simulink model "CAProcessorInTheLoop"  (R2022b)
settings: Solver=FixedStepAuto  StartTime=0.0  StopTime=100.0  RelTol=1e-3  EnableMultiTasking=on
InitFcn:
  | init_fn()
values from neighbouring files (symbols this model uses):
  X_air = evalin('base', 'X_air')    [init_fn.m]
undefined symbols (not defined in the file or in its folder): m, MAX_SPEED_BACKWARD, MAX_SPEED_FORWARD, MAX_TORQUE, MAX_TORQUE_REVERSE, r, TRANSMISSION_RATIO, X_tyres
libraries: arduinolib x25, slpidlib x1
settings Model: ExtModeTrigDuration=2  Creator=David  LastModifiedBy=David
settings OptimizationCC: EnhancedBackFolding=on  PassReuseOutputArgsAs=Individual arguments  ZeroExternalMemoryAtStartup=off  ZeroInternalMemoryAtStartup=off  MaxStackSize=64  OptimizeBlockOrder=speed  DifferentSizesBufferReuse=on  OptimizationCustomize=off  EfficientTunableParamExpr=on
settings DebuggingCC: ParameterOverflowMsg=none  ParameterUnderflowMsg=error  ParameterPrecisionLossMsg=none  ParameterTunabilityLossMsg=error
settings HardwareCC: ProdBitPerInt=16  ProdBitPerPointer=16  ProdBitPerSizeT=16  ProdBitPerPtrDiffT=16  ProdLargestAtomicFloat=None  ProdWordSize=8  ProdHWDeviceType=Atmel->AVR
settings SFSimCC: MATLABDynamicMemAlloc=off
settings RTWCC: Description=Embedded Coder  SystemTargetFile=ert.tlc  HardwareBoard=Arduino Mega 2560  TLCOptions=-aInlineSetEventsForThisBaseRateFcn=TLC_FALSE -aSuppressMultiTaskScheduler=TLC_FALSE -aRateBasedStepFcn=1  TemplateMakefile=ert_default_tmf  Toolchain=Arduino AVR
settings CodeAppCC: ForceParamTrailComments=on  IgnoreCustomStorageClasses=off  OperatorAnnotations=on  SimulinkDataObjDesc=on  SFDataObjDesc=on  InsertBlockDesc=on
settings ERTTargetCC: SupportContinuousTime=on  SupportVariableSizeSignals=on  ExtModeTransport=3  ExtModeStaticAlloc=on  ExtModeAutomaticAllocSize=off  ExtModeStaticAllocSize=2048  ExtModeMexFile=ext_xcp  ExtModeIntrfLevel=Level2 - Open

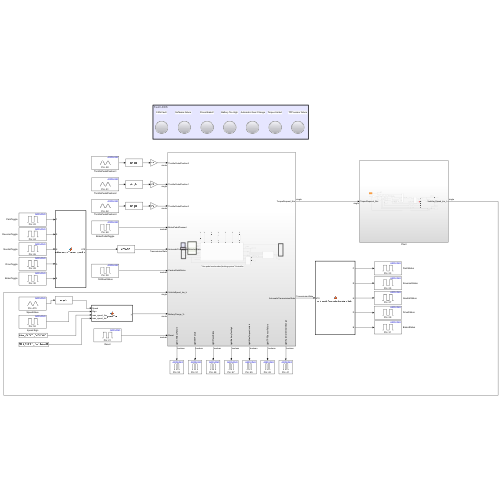
[thumbnail: Simulink's stored preview of the top-level diagram]
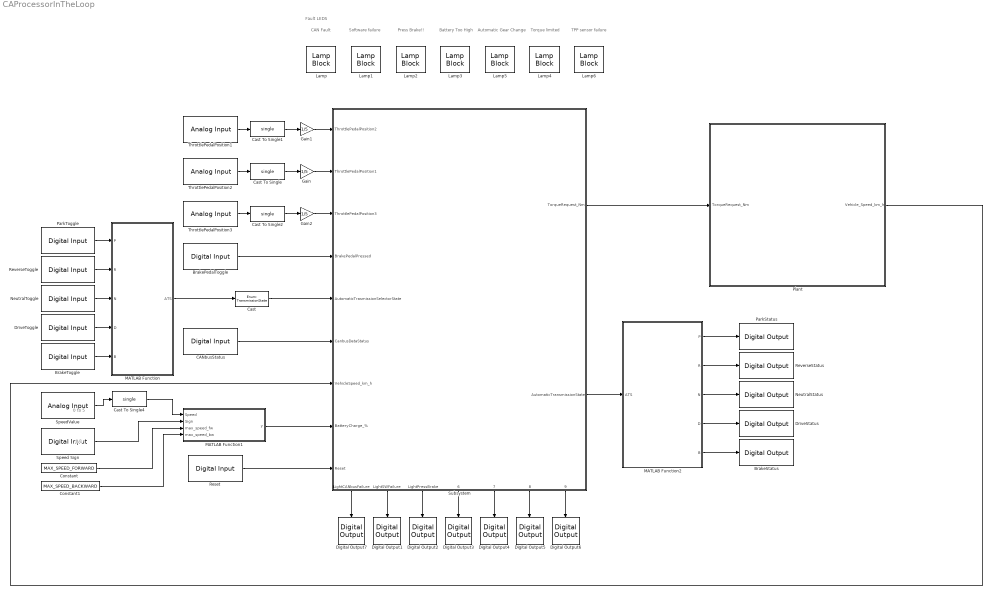
== system CAProcessorInTheLoop ==
  note: Fault LEDS
  note: 0 to 5
  note: CAN Fault
  note: Automatic Gear Change
  note: Press Brake!!
  note: Battery Too High
  note: Software failure
  note: TPP sensor failure
  note: Torque limited
  note: 0/1
  BrakePedalToggle : arduinolib/Digital Input  pinNumber=48  mode=Default  Direction=input  SampleTime=0.01  blockPlatform=arduino
  BrakeStatus : arduinolib/Digital Output  pinNumber=31  Direction=output  blockPlatform=arduino
  BrakeToggle : arduinolib/Digital Input  pinNumber=30  mode=Default  Direction=input  SampleTime=0.01  blockPlatform=arduino
  CANbusStatus : arduinolib/Digital Input  pinNumber=50  mode=Default  Direction=input  SampleTime=0.01  blockPlatform=arduino
  Cast : DataTypeConversion  OutDataTypeStr=Enum: TransmissionState  SaturateOnIntegerOverflow=off  RndMeth=Floor
  Cast To Single{,1..2,4} (4 alike) : DataTypeConversion  OutDataTypeStr=single  SaturateOnIntegerOverflow=off  RndMeth=Floor
  Constant : Constant  Value=MAX_SPEED_FORWARD  OutDataTypeStr=single
  Constant1 : Constant  Value=MAX_SPEED_BACKWARD  OutDataTypeStr=single
  Digital Output1 : arduinolib/Digital Output  pinNumber=51  Direction=output  blockPlatform=arduino
  Digital Output2 : arduinolib/Digital Output  pinNumber=49  Direction=output  blockPlatform=arduino
  Digital Output3 : arduinolib/Digital Output  pinNumber=47  Direction=output  blockPlatform=arduino
  Digital Output4 : arduinolib/Digital Output  pinNumber=45  Direction=output  blockPlatform=arduino
  Digital Output5 : arduinolib/Digital Output  pinNumber=43  Direction=output  blockPlatform=arduino
  Digital Output6 : arduinolib/Digital Output  pinNumber=41  Direction=output  blockPlatform=arduino
  Digital Output7 : arduinolib/Digital Output  pinNumber=53  Direction=output  blockPlatform=arduino
  DriveStatus : arduinolib/Digital Output  pinNumber=29  Direction=output  blockPlatform=arduino
  DriveToggle : arduinolib/Digital Input  pinNumber=28  mode=Default  Direction=input  SampleTime=0.01  blockPlatform=arduino
  Gain : Gain  Gain=1/5
  Gain1 : Gain  Gain=1/5
  Gain2 : Gain  Gain=1/5
  Lamp{,1..6} (7 alike) : LampBlock  LabelPosition=Hide
  MATLAB Function : MATLAB Function  TreatAsAtomicUnit=on
  MATLAB Function1 : MATLAB Function  TreatAsAtomicUnit=on
  MATLAB Function2 : MATLAB Function  TreatAsAtomicUnit=on
  NeutralStatus : arduinolib/Digital Output  pinNumber=27  Direction=output  blockPlatform=arduino
  NeutralToggle : arduinolib/Digital Input  pinNumber=26  mode=Default  Direction=input  SampleTime=0.01  blockPlatform=arduino
  ParkStatus : arduinolib/Digital Output  pinNumber=23  Direction=output  blockPlatform=arduino
  ParkToggle : arduinolib/Digital Input  pinNumber=22  mode=Default  Direction=input  SampleTime=0.01  blockPlatform=arduino
  Plant : Subsystem
  Reset : arduinolib/Digital Input  pinNumber=21  mode=Default  Direction=input  SampleTime=0.01  blockPlatform=arduino
  ReverseStatus : arduinolib/Digital Output  pinNumber=25  Direction=output  blockPlatform=arduino
  ReverseToggle : arduinolib/Digital Input  pinNumber=24  mode=Default  Direction=input  SampleTime=0.01  blockPlatform=arduino
  Speed Sign : arduinolib/Digital Input  pinNumber=52  mode=Default  Direction=input  SampleTime=0.01  blockPlatform=arduino
  SpeedValue : arduinolib/Analog Input  pinNumber=15  ReadResultsOnly=off  ConversionTriggerSource=Software  ExternalTriggerType=uint32( 0 )  OutputDataType=uint16  EnableConversionCompleteNotify=off  EnableOuputStatus=off  SampleTime=-1  blockPlatform=arduino
  Subsystem : Subsystem
      settings: PortSchema="{\"entries\":[{\"content\":{\"sides\":[{\"content\":{\"connectorIds\":[\"In1\",\"In2\",\"In3\",\"In4\",\"In5\",\"In6\",\"In7\",\"In8\",\"In9\"]},\"type\":\"ConnectorPlacement.EquallySpacedRectSide\",\"uuid\":\"240cc9ec-2ba8-4d42-9768-bf8b5b2cd18c\"},{\"content\":{\"connectorIds\":[\"Out1\",\"Out2\"],\"side\":\"RIGHT\"},\"type\":\"ConnectorPlacement.EquallySpacedRectSide\",\"uuid\":\"79e5a8d1-1f90-4926-ab4a-0fddf072b8d0\"},{\"content\":{\"connectorIds\":[],\"side\":\"TOP\"},\"type\":\"ConnectorPlacement.EquallySpacedRectSide\",\"uuid\":\"0e8827e4-c087-4ef4-9de2-35b882084602\"},{\"content\":{\"connectorIds\":[\"Out3\",\"Out4\",\"Out5\",\"Out6\",\"Out7\",\"Out8\",\"Out9\"],\"side\":\"BOTTOM\"},\"type\":\"ConnectorPlacement.EquallySpacedRectSide\",\"uuid\":\"1cd7cba7-84b1-4c6c-afc4-562411f8f962\"}]},\"type\":\"ConnectorPlacement.EquallySpacedConnector\",\"uuid\":\"eda7bf13-88b7-423b-9505-3784a3aa3e13\"}],\"packageUris\":[\"http://schema.mathworks.com/mf0/Connector/R2020b\"],\"version\":\"1.0\"}"
  ThrottlePedalPosition1 : arduinolib/Analog Input  pinNumber=0  ReadResultsOnly=off  ConversionTriggerSource=Software  ExternalTriggerType=uint32( 0 )  OutputDataType=uint16  EnableConversionCompleteNotify=off  EnableOuputStatus=off  SampleTime=-1  blockPlatform=arduino
  ThrottlePedalPosition2 : arduinolib/Analog Input  pinNumber=1  ReadResultsOnly=off  ConversionTriggerSource=Software  ExternalTriggerType=uint32( 0 )  OutputDataType=uint16  EnableConversionCompleteNotify=off  EnableOuputStatus=off  SampleTime=-1  blockPlatform=arduino
  ThrottlePedalPosition3 : arduinolib/Analog Input  pinNumber=2  ReadResultsOnly=off  ConversionTriggerSource=Software  ExternalTriggerType=uint32( 0 )  OutputDataType=uint16  EnableConversionCompleteNotify=off  EnableOuputStatus=off  SampleTime=-1  blockPlatform=arduino
  wires:
  ThrottlePedalPosition2/1 -> Cast To Single/1
  Gain/1 -> Subsystem/2(ThrottlePedalPosition1)
  Gain1/1 -> Subsystem/1(ThrottlePedalPosition2)
  ThrottlePedalPosition1/1 -> Cast To Single1/1
  Gain2/1 -> Subsystem/3(ThrottlePedalPosition3)
  ThrottlePedalPosition3/1 -> Cast To Single2/1
  ParkToggle/1 -> MATLAB Function/1(P)
  ReverseToggle/1 -> MATLAB Function/2(R)
  NeutralToggle/1 -> MATLAB Function/3(N)
  DriveToggle/1 -> MATLAB Function/4(D)
  CANbusStatus/1 -> Subsystem/6(CanbusDataStatus)
  SpeedValue/1 -> Cast To Single4/1
  MATLAB Function1/1(y) -> Subsystem/8(BatteryCharge_%)
  Speed Sign/1 -> MATLAB Function1/2(Sign)
  Subsystem/2(AutomaticTransmissionState) -> MATLAB Function2/1(ATS)
  MATLAB Function2/1(P) -> ParkStatus/1
  MATLAB Function2/2(R) -> ReverseStatus/1
  MATLAB Function2/3(N) -> NeutralStatus/1
  MATLAB Function2/4(D) -> DriveStatus/1
  MATLAB Function2/5(B) -> BrakeStatus/1
  Subsystem/1(TorqueRequest_Nm) -> Plant/1(TorqueRequest_Nm)
  Cast To Single/1 -> Gain/1
  Cast To Single1/1 -> Gain1/1
  Cast To Single2/1 -> Gain2/1
  Cast To Single4/1 -> MATLAB Function1/1(Speed)
  Constant/1 -> MATLAB Function1/3(max_speed_fw)
  Constant1/1 -> MATLAB Function1/4(max_speed_bw)
  Cast/1 -> Subsystem/5(AutomaticTrasmissionSelectorState)
  MATLAB Function/1(ATS) -> Cast/1
  BrakePedalToggle/1 -> Subsystem/4(BrakePedalPressed)
  BrakeToggle/1 -> MATLAB Function/5(B)
  Subsystem/3(LightCANbusFailure) -> Digital Output7/1
  Subsystem/4(LightSWFailure) -> Digital Output1/1
  Subsystem/5(LightPressBrake) -> Digital Output2/1
  Subsystem/6(LightBatteryTooHigh) -> Digital Output3/1
  Subsystem/7(LightMaxTorqueLimited) -> Digital Output4/1
  Subsystem/8(LightTPPSensorFailure) -> Digital Output5/1
  Subsystem/9(LightAutomaticGearChange) -> Digital Output6/1
  Reset/1 -> Subsystem/9(Reset)
  Plant/1(Vehicle_Speed_km_h) -> Subsystem/7(VehicleSpeed_km_h)

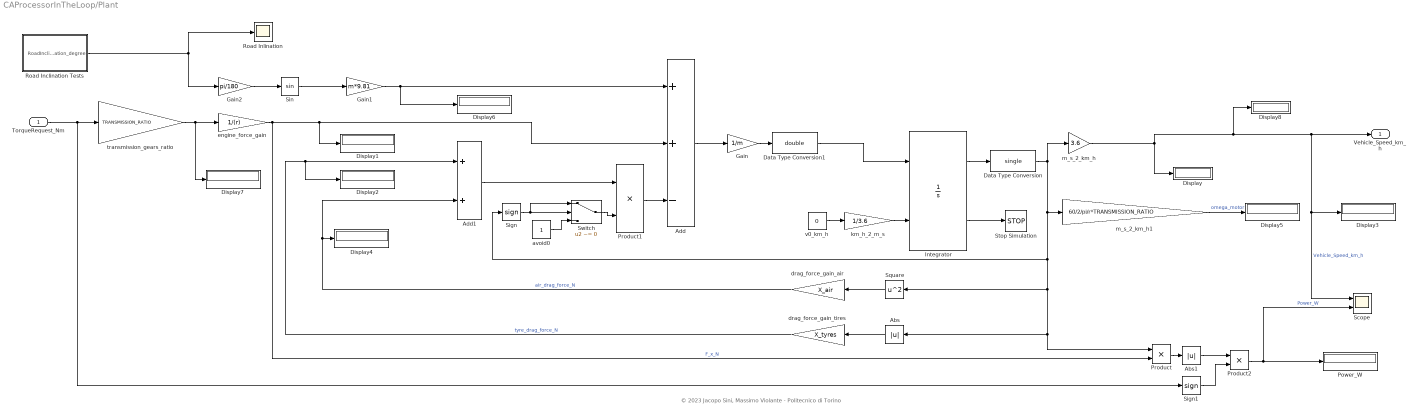
== system CAProcessorInTheLoop/Plant ==
  note: © 2023 Jacopo Sini, Massimo Violante - Politecnico di Torino
  TorqueRequest_Nm : Inport  OutDataTypeStr=single
  Abs : Abs  SaturateOnIntegerOverflow=off
  Abs1 : Abs  SaturateOnIntegerOverflow=off
  Add : Sum  Inputs=++-
  Add1 : Sum
  Data Type Conversion : DataTypeConversion  OutDataTypeStr=single  SaturateOnIntegerOverflow=off  RndMeth=Floor  LockScale=on
  Data Type Conversion1 : DataTypeConversion  OutDataTypeStr=double  SaturateOnIntegerOverflow=off  RndMeth=Floor  LockScale=on
  Display{,1..8} (9 alike) : Display
      Display1 settings: Format=bank
      Display2 settings: Format=bank
      Display3 settings: Format=bank
      Display4 settings: Format=bank
      Display5 settings: Format=bank
      Display6 settings: Format=bank
      Display7 settings: Format=bank
  Gain : Gain  Gain=1/m
  Gain1 : Gain  Gain=m*9.81
  Gain2 : Gain  Gain=pi/180
  Integrator : Integrator  InitialConditionSource=external  LimitOutput=on  UpperSaturationLimit=MAX_SPEED_FORWARD/3.6  LowerSaturationLimit=-MAX_SPEED_BACKWARD/3.6  ShowSaturationPort=on  ContinuousStateAttributes='vehicle_speed'
  Power_W : Display
      settings: Format=bank
  Product : Product
  Product1 : Product
  Product2 : Product
  Road Inclination Tests : Subsystem
  Road Inlination : Scope
  Scope : Scope  NumInputPorts=2
  Sign : Signum  ZeroCross=off
  Sign1 : Signum  ZeroCross=off
  Sin : Trigonometry  OutputSignalType=real
  Square : Math  Operator=square
  Stop Simulation : Stop
  Switch : Switch  Criteria=u2 ~= 0  SaturateOnIntegerOverflow=off  InputSameDT=off
  avoid0 : Constant  OutDataTypeStr=double
  drag_force_gain_air : Gain  Gain=X_air
  drag_force_gain_tires : Gain  Gain=X_tyres
  engine_force_gain : Gain  Gain=1/(r)
  km_h_2_m_s : Gain  Gain=1/3.6
  m_s_2_km_h : Gain  Gain=3.6
  m_s_2_km_h1 : Gain  Gain=60/2/pi/r*TRANSMISSION_RATIO
  transmission_gears_ratio : Gain  Gain=TRANSMISSION_RATIO
  v0_km_h : Constant  Value=0  OutDataTypeStr=double
  Vehicle_Speed_km_h : Outport  OutDataTypeStr=single  Unit=km/h
  wires:
  TorqueRequest_Nm/1 -> Sign1/1, transmission_gears_ratio/1
  Add1/1 -> Product1/1
  Square/1 -> drag_force_gain_air/1
  Data Type Conversion1/1 -> Integrator/1
  v0_km_h/1 -> km_h_2_m_s/1
  Product1/1 -> Add/3
  engine_force_gain/1 -> Product/2, Display1/1, Add/2  "F_x_N"
  Sign/1 -> Switch/1, Switch/2
  Abs/1 -> drag_force_gain_tires/1
  Sign1/1 -> Product2/2
  Abs1/1 -> Product2/1
  km_h_2_m_s/1 -> Integrator/2
  Gain1/1 -> Display6/1, Add/1
  Product2/1 -> Scope/2, Power_W/1  "Power_W"
  Integrator/1 -> Data Type Conversion/1
  drag_force_gain_tires/1 -> Display2/1, Add1/1  "tyre_drag_force_N"
  Sin/1 -> Gain1/1
  Product/1 -> Abs1/1
  Data Type Conversion/1 -> Sign/1, Product/1, Abs/1, Square/1, m_s_2_km_h1/1, m_s_2_km_h/1
  transmission_gears_ratio/1 -> engine_force_gain/1, Display7/1
  avoid0/1 -> Switch/3
  Switch/1 -> Product1/2
  Road Inclination Tests/1(RoadInclination_degree) -> Road Inlination/1, Gain2/1
  Gain2/1 -> Sin/1
  drag_force_gain_air/1 -> Add1/2, Display4/1  "air_drag_force_N"
  Gain/1 -> Data Type Conversion1/1
  Add/1 -> Gain/1
  m_s_2_km_h/1 -> Display8/1, Scope/1, Display3/1, Vehicle_Speed_km_h/1, Display/1  "Vehicle_Speed_km_h"
  Integrator/2 -> Stop Simulation/1
  m_s_2_km_h1/1 -> Display5/1  "omega_motor"

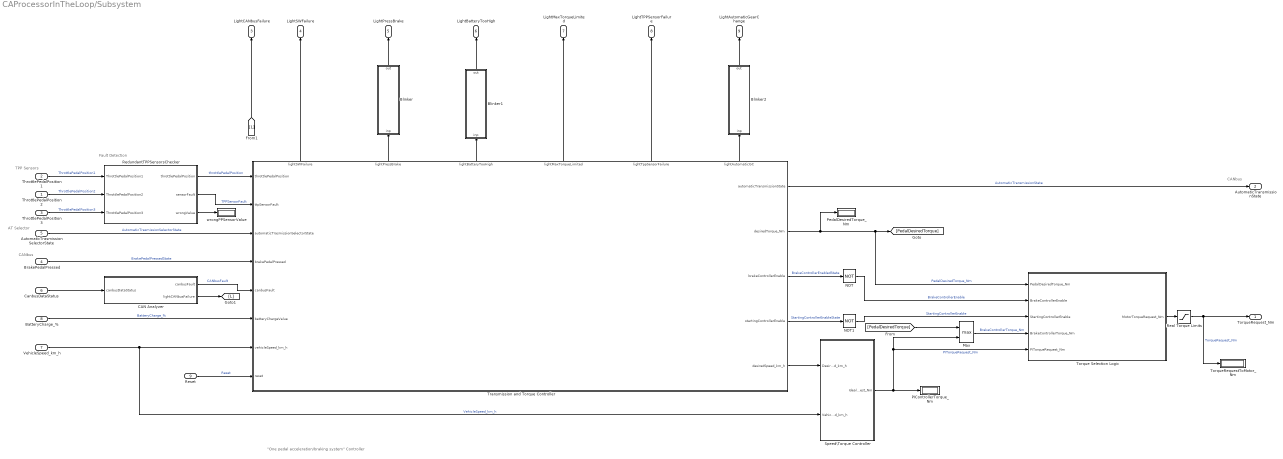
== system CAProcessorInTheLoop/Subsystem ==
  note: TPP Sensors
  note: CANbus
  note: "One pedal acceleration/braking system" Controller
  note: Fault Detection
  note: AT Selector
  note: CANbus
  ThrottlePedalPosition2 : Inport  OutDataTypeStr=single
  ThrottlePedalPosition1 : Inport  Port=2  OutDataTypeStr=single
  ThrottlePedalPosition3 : Inport  Port=3  OutDataTypeStr=single
  BrakePedalPressed : Inport  Port=4  OutDataTypeStr=boolean
  AutomaticTrasmissionSelectorState : Inport  Port=5  OutDataTypeStr=Enum: TransmissionState
  CanbusDataStatus : Inport  Port=6  OutDataTypeStr=boolean  Unit=km/h
  VehicleSpeed_km_h : Inport  Port=7  OutDataTypeStr=single  Unit=km/h
  BatteryCharge_% : Inport  Port=8  OutDataTypeStr=single  Unit=km/h
  Reset : Inport  Port=9  OutDataTypeStr=boolean  Unit=km/h
  Blinker : Stateflow chart  TreatAsAtomicUnit=on
  Blinker1 : Stateflow chart  TreatAsAtomicUnit=on
  Blinker2 : Stateflow chart  TreatAsAtomicUnit=on
  CAN Analyzer : Stateflow chart  TreatAsAtomicUnit=on
  Max : MinMax  Function=max  Inputs=2
  NOT : Logic  Operator=NOT  IconShape=distinctive  AllPortsSameDT=off  OutDataTypeStr=boolean
  NOT1 : Logic  Operator=NOT  IconShape=distinctive  AllPortsSameDT=off  OutDataTypeStr=boolean
  PIControllerTorque_Nm : Display
  PedalDesiredTorque_Nm : Display
  Real Torque Limits : Saturate  UpperLimit=MAX_TORQUE  LowerLimit=-MAX_TORQUE_REVERSE
  RedundantTPPSensorsChecker : Subsystem
  Speed\Torque Controller : Subsystem
  Torque Selection Logic : Subsystem
  TorqueRequestToMotor_Nm : Display
  Transmission and Torque Controller : Stateflow chart  TreatAsAtomicUnit=on
      settings: PortSchema="{\"entries\":[{\"content\":{\"sides\":[{\"content\":{\"connectorIds\":[\"In1\",\"In2\",\"In4\",\"In3\",\"In5\",\"In6\",\"In7\",\"In8\"]},\"type\":\"ConnectorPlacement.EquallySpacedRectSide\",\"uuid\":\"0c8aad20-bedd-441c-a5c9-bebe8b868021\"},{\"content\":{\"connectorIds\":[\"Out1\",\"Out2\",\"Out3\",\"Out4\",\"Out5\"],\"side\":\"RIGHT\"},\"type\":\"ConnectorPlacement.EquallySpacedRectSide\",\"uuid\":\"1881f9b3-9ea6-444d-9c49-eff5d4926a82\"},{\"content\":{\"connectorIds\":[\"Out6\",\"Out7\",\"Out8\",\"Out9\",\"Out10\",\"Out11\"],\"side\":\"TOP\"},\"type\":\"ConnectorPlacement.EquallySpacedRectSide\",\"uuid\":\"de055a5d-6f50-4d63-823e-754d8458ae2a\"}]},\"type\":\"ConnectorPlacement.EquallySpacedConnector\",\"uuid\":\"28ac9a9c-8f29-4c5e-bfec-f6af3b41ee50\"}],\"packageUris\":[\"http://schema.mathworks.com/mf0/Connector/R2020b\"],\"version\":\"1.0\"}"
  wrongPPSensorValue : Display
  TorqueRequest_Nm : Outport  OutDataTypeStr=single  Unit=N*m
  AutomaticTransmissionState : Outport  Port=2  OutDataTypeStr=Enum: TransmissionState
  LightCANbusFailure : Outport  Port=3  OutDataTypeStr=boolean
  LightSWFailure : Outport  Port=4  OutDataTypeStr=boolean
  LightPressBrake : Outport  Port=5  OutDataTypeStr=boolean
  LightBatteryTooHigh : Outport  Port=6  OutDataTypeStr=boolean
  LightMaxTorqueLimited : Outport  Port=7  OutDataTypeStr=boolean
  LightTPPSensorFailure : Outport  Port=8  OutDataTypeStr=boolean
  LightAutomaticGearChange : Outport  Port=9  OutDataTypeStr=boolean
  wires:
  ThrottlePedalPosition1/1 -> RedundantTPPSensorsChecker/1(ThrottlePedalPosition1)  "ThrottlePedalPosition1"
  ThrottlePedalPosition2/1 -> RedundantTPPSensorsChecker/2(ThrottlePedalPosition2)  "ThrottlePedalPosition2"
  Transmission and Torque Controller/6(lightSWFailure) -> LightSWFailure/1
  CanbusDataStatus/1 -> CAN Analyzer/1(canbusDataStatus)
  Transmission and Torque Controller/11(lightAutomaticGC) -> Blinker2/1(inp)
  [L] -> LightCANbusFailure/1
  ThrottlePedalPosition3/1 -> RedundantTPPSensorsChecker/3(ThrottlePedalPosition3)  "ThrottlePedalPosition3"
  Transmission and Torque Controller/7(lightPressBrake) -> Blinker/1(inp)
  AutomaticTrasmissionSelectorState/1 -> Transmission and Torque Controller/4(automaticTrasmissionSelectorState)  "AutomaticTrasmissionSelectorState"
  [PedalDesiredTorque] -> Max/1
  Blinker2/1(out) -> LightAutomaticGearChange/1
  Reset/1 -> Transmission and Torque Controller/8(reset)  "Reset"
  Transmission and Torque Controller/10(lightTppSensorFailure) -> LightTPPSensorFailure/1
  Blinker/1(out) -> LightPressBrake/1
  NOT1/1 -> Torque Selection Logic/3(StartingControllerEnable)  "StartingControllerEnable"
  NOT/1 -> Torque Selection Logic/2(BrakeControllerEnable)  "BrakeControllerEnable"
  Torque Selection Logic/1(MotorTorqueRequest_Nm) -> Real Torque Limits/1
  RedundantTPPSensorsChecker/3(wrongValue) -> wrongPPSensorValue/1
  Transmission and Torque Controller/2(desiredTorque_Nm) -> PedalDesiredTorque_Nm/1, [PedalDesiredTorque], Torque Selection Logic/1(PedalDesiredTorque_Nm)  "PedalDesiredTorque_Nm"
  CAN Analyzer/2(lightCANbusFailure) -> [L]
  BrakePedalPressed/1 -> Transmission and Torque Controller/3(brakePedalPressed)  "BrakePedalPressedState"
  Transmission and Torque Controller/3(brakeControllerEnable) -> NOT/1  "BrakeControllerEnabledState"
  CAN Analyzer/1(canbusFault) -> Transmission and Torque Controller/5(canbusFault)  "CANbusFault"
  RedundantTPPSensorsChecker/1(throttlePedalPosition) -> Transmission and Torque Controller/1(throttlePedalPosition)  "throttlePedalPosition"
  Transmission and Torque Controller/1(automaticTransmissionState) -> AutomaticTransmissionState/1  "AutomaticTransmissionState"
  BatteryCharge_%/1 -> Transmission and Torque Controller/6(batteryChargeValue)  "BatteryCharge_%"
  Blinker1/1(out) -> LightBatteryTooHigh/1
  VehicleSpeed_km_h/1 -> Transmission and Torque Controller/7(vehicleSpeed_km_h), Speed\Torque Controller/2(VehicleSpeed_km_h)  "VehicleSpeed_km_h"
  Transmission and Torque Controller/8(lightBatteryTooHigh) -> Blinker1/1(inp)
  Speed\Torque Controller/1(IdealTorqueRequest_Nm) -> PIControllerTorque_Nm/1, Torque Selection Logic/5(PITorqueRequest_Nm), Max/2  "PITorqueRequest_Nm"
  Max/1 -> Torque Selection Logic/4(BrakeControllerTorque_Nm)  "BrakeControllerTorque_Nm"
  Transmission and Torque Controller/5(desiredSpeed_km_h) -> Speed\Torque Controller/1(DesiredSpeed_km_h)
  RedundantTPPSensorsChecker/2(sensorFault) -> Transmission and Torque Controller/2(ttpSensorFault)  "TPPSensorFault"
  Transmission and Torque Controller/9(lightMaxTorqueLimited) -> LightMaxTorqueLimited/1
  Transmission and Torque Controller/4(startingControllerEnable) -> NOT1/1  "StartingControllerEnableState"
  Real Torque Limits/1 -> TorqueRequest_Nm/1, TorqueRequestToMotor_Nm/1  "TorqueRequest_Nm"

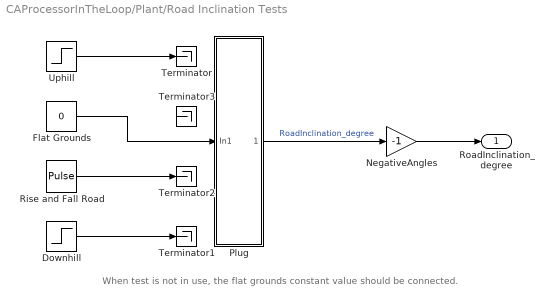
== system CAProcessorInTheLoop/Plant/Road Inclination Tests ==
  note: When test is not in use, the flat grounds constant value should be connected.
  Downhill : Step  Time=3  After=-4  SampleTime=0
  Flat Grounds : Constant  Value=0
  NegativeAngles : Gain  Gain=-1
  Plug : Subsystem
  Rise and Fall Road : DiscretePulseGenerator  PulseType=Time based  Amplitude=0  PulseWidth=50  PhaseDelay=5
  Terminator{,1..3} (4 alike) : Terminator
  Uphill : Step  Time=30  After=10  SampleTime=0
  RoadInclination_degree : Outport
  wires:
  NegativeAngles/1 -> RoadInclination_degree/1
  Plug/1(Out1) -> NegativeAngles/1  "RoadInclination_degree"
  Downhill/1 -> Terminator1/1
  Rise and Fall Road/1 -> Terminator2/1
  Uphill/1 -> Terminator/1
  Flat Grounds/1 -> Plug/1(In1)

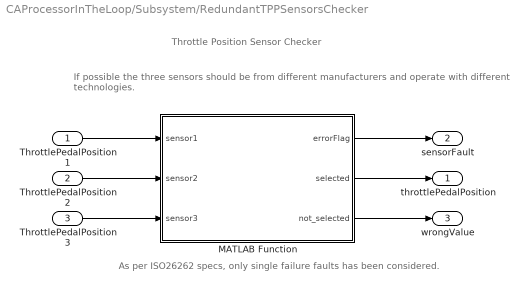
== system CAProcessorInTheLoop/Subsystem/RedundantTPPSensorsChecker ==
  note: As per ISO26262 specs, only single failure faults has been considered.
  note: Throttle Position Sensor Checker
  note: If possible the three sensors should be from different manufacturers and operate with different technologies.
  ThrottlePedalPosition1 : Inport
  ThrottlePedalPosition2 : Inport  Port=2
  ThrottlePedalPosition3 : Inport  Port=3
  MATLAB Function : MATLAB Function  TreatAsAtomicUnit=on
  throttlePedalPosition : Outport
  sensorFault : Outport  Port=2  OutDataTypeStr=boolean
  wrongValue : Outport  Port=3
  wires:
  ThrottlePedalPosition1/1 -> MATLAB Function/1(sensor1)
  ThrottlePedalPosition3/1 -> MATLAB Function/3(sensor3)
  ThrottlePedalPosition2/1 -> MATLAB Function/2(sensor2)
  MATLAB Function/1(errorFlag) -> sensorFault/1
  MATLAB Function/2(selected) -> throttlePedalPosition/1
  MATLAB Function/3(not_selected) -> wrongValue/1

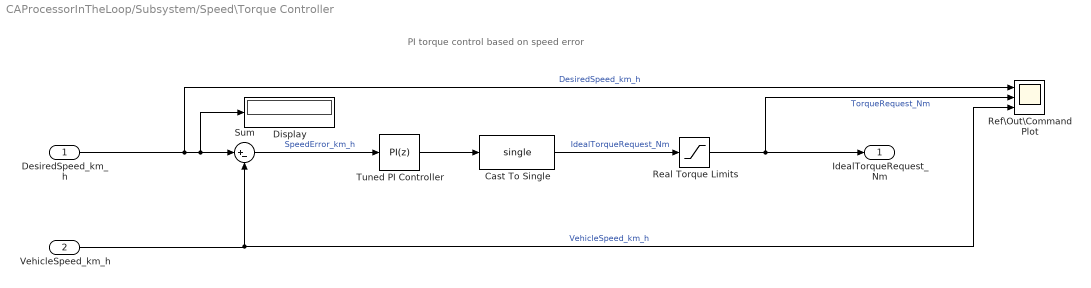
== system CAProcessorInTheLoop/Subsystem/Speed\Torque Controller ==
  note: PI torque control based on speed error
  DesiredSpeed_km_h : Inport
  VehicleSpeed_km_h : Inport  Port=2
  Cast To Single : DataTypeConversion  OutDataTypeStr=single  SaturateOnIntegerOverflow=off  RndMeth=Floor
  Display : Display
  Real Torque Limits : Saturate  UpperLimit=MAX_TORQUE  LowerLimit=-MAX_TORQUE_REVERSE
  Ref\Out\Command Plot : Scope  NumInputPorts=3
  Sum : Sum  Inputs=|+-
  Tuned PI Controller : slpidlib/PID Controller  Controller=PI  Form=Parallel  TimeDomain=Discrete-time  UseExternalTs=off  SampleTime=1/100  IntegratorMethod=Forward Euler  FilterMethod=Forward Euler  ControllerParametersSource=internal  P=79.689863897109  I=82.1622460012644  UseKiTs=off  D=2.01264569507152  N=1.91388047645984  UseFilter=on  TunerSelectOption=Transfer Function Based (PID Tuner App)  InitialConditionSource=internal  InitialConditionForIntegrator=0  InitialConditionForFilter=0  DifferentiatorICPrevScaledInput=0  ExternalReset=none  TrackingMode=off  Kt=1  LimitOutput=off  SatLimitsSource=internal  UpperSaturationLimit=MAX_TORQUE  LowerSaturationLimit=-MAX_TORQUE_REVERSE  LinearizeAsGain=on  AntiWindupMode=none  Kb=1  LimitIntegrator=on  UpperIntegratorSaturationLimit=MAX_TORQUE  LowerIntegratorSaturationLimit=-MAX_TORQUE_REVERSE  POutMin=[]  POutMax=[]  IOutMin=[]  IOutMax=[]  DOutMin=[]  DOutMax=[]  NOutMin=[]  NOutMax=[]  SumOutMin=[]  SumOutMax=[]  SaturationOutMin=[]  SaturationOutMax=[]  PParamMin=[]  PParamMax=[]  IParamMin=[]  IParamMax=[]  DParamMin=[]  DParamMax=[]  NParamMin=[]  NParamMax=[]  KbParamMin=[]  KbParamMax=[]  KtParamMin=[]  KtParamMax=[]  KbOutMin=[]  KbOutMax=[]  KtOutMin=[]  KtOutMax=[]  IntegratorOutMin=[]  IntegratorOutMax=[]  FilterOutMin=[]  FilterOutMax=[]  SumI1OutMin=[]  SumI1OutMax=[]  SumI2OutMin=[]  SumI2OutMax=[]  SumI3OutMin=[]  SumI3OutMax=[]  SumI4OutMin=[]  SumI4OutMax=[]  SumDOutMin=[]  SumDOutMax=[]  DifferentiatorOutMin=[]  DifferentiatorOutMax=[]  FilterDiffOutCoefMin=[]  FilterDiffOutCoefMax=[]  ReciprocalOutMin=[]  ReciprocalOutMax=[]  SumDenOutMin=[]  SumDenOutMax=[]  SumNumOutMin=[]  SumNumOutMax=[]  DivideOutMin=[]  DivideOutMax=[]  UdiffTsProdOutMin=[]  UdiffTsProdOutMax=[]  NTsProdOutMin=[]  NTsProdOutMax=[]  UintegralTsProdOutMin=[]  UintegralTsProdOutMax=[]  UngainTsProdOutMin=[]  UngainTsProdOutMax=[]  ClampingZeroOutDataTypeStr=Inherit: Inherit via back propagation  ClampingZeroOutMin=[]  ClampingZeroOutMax=[]  FilterDenConstantOutDataTypeStr=Inherit: Inherit via back propagation  FilterDenConstantOutMin=[]  FilterDenConstantOutMax=[]  PCopyOutDataTypeStr=Inherit: Inherit via back propagation  PCopyOutMin=[]  PCopyOutMax=[]  NCopyOutDataTypeStr=Inherit: Inherit via back propagation  NCopyOutMin=[]  NCopyOutMax=[]  IntegratorContinuousStateAttributes=''  IntegratorStateMustResolveToSignalObject=off  IntegratorRTWStateStorageClass=Auto  FilterContinuousStateAttributes=''  FilterStateMustResolveToSignalObject=off  FilterRTWStateStorageClass=Auto  ParallelPVariant=InternalParameters  IdealPVariant=Disabled  IVariant=InternalParameters  DVariant=Disabled  IntegratorVariant=Discrete  SatVariant=Disabled  AWVariant=Passthrough  PCopyVariant=Disabled  TRVariant=Disabled  FdbkBlocksVariant=Forward  IdealPFdbkVariant=Disabled  SatFdbkVariant=Disabled  DerivativeFilterVariant=Disabled  NVariant=Disabled  NCopyVariant=Disabled_SignalSpec  FilterICVariant=Disabled  IntegratorICVariant=InternalICs  ExternalResetVariant=Disabled  TRSumVariant=Passthrough  SumFdbkVariant=Disabled  SumVariant=Sum_PI  TsampFilterVariant=InternalTs  TsampNgainVariant=Passthrough  TsampIntegralVariant=Passthrough  ExternalSaturationOutDataTypeStr=Inherit: Same as second input
  IdealTorqueRequest_Nm : Outport
  wires:
  Cast To Single/1 -> Real Torque Limits/1  "IdealTorqueRequest_Nm"
  Tuned PI Controller/1 -> Cast To Single/1
  DesiredSpeed_km_h/1 -> Ref\Out\Command Plot/1, Display/1, Sum/1  "DesiredSpeed_km_h"
  VehicleSpeed_km_h/1 -> Ref\Out\Command Plot/3, Sum/2  "VehicleSpeed_km_h"
  Sum/1 -> Tuned PI Controller/1  "SpeedError_km_h"
  Real Torque Limits/1 -> Ref\Out\Command Plot/2, IdealTorqueRequest_Nm/1  "TorqueRequest_Nm"

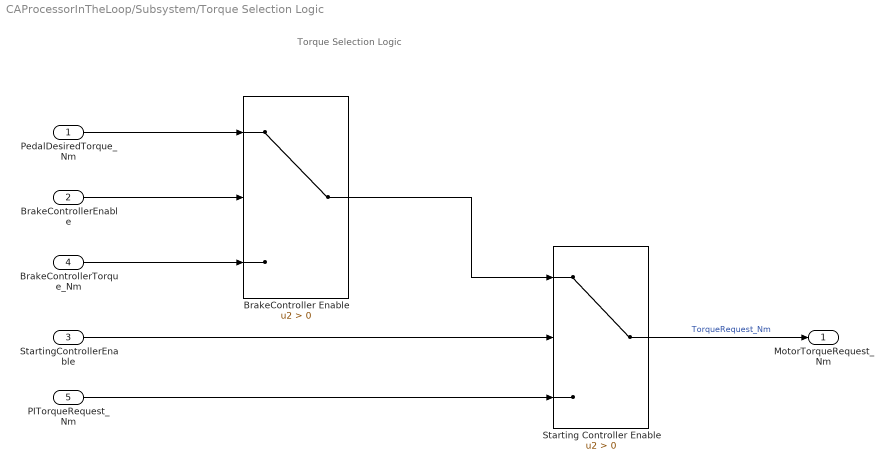
== system CAProcessorInTheLoop/Subsystem/Torque Selection Logic ==
  note: Torque Selection Logic
  PedalDesiredTorque_Nm : Inport
  BrakeControllerEnable : Inport  Port=2
  StartingControllerEnable : Inport  Port=3
  BrakeControllerTorque_Nm : Inport  Port=4
  PITorqueRequest_Nm : Inport  Port=5
  BrakeController Enable : Switch  Criteria=u2 > Threshold  SaturateOnIntegerOverflow=off  InputSameDT=off
  Starting Controller Enable : Switch  Criteria=u2 > Threshold  SaturateOnIntegerOverflow=off  InputSameDT=off
  MotorTorqueRequest_Nm : Outport
  wires:
  StartingControllerEnable/1 -> Starting Controller Enable/2
  BrakeControllerEnable/1 -> BrakeController Enable/2
  BrakeController Enable/1 -> Starting Controller Enable/1
  BrakeControllerTorque_Nm/1 -> BrakeController Enable/3
  Starting Controller Enable/1 -> MotorTorqueRequest_Nm/1  "TorqueRequest_Nm"
  PITorqueRequest_Nm/1 -> Starting Controller Enable/3
  PedalDesiredTorque_Nm/1 -> BrakeController Enable/1

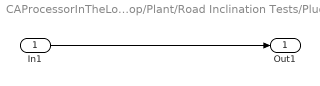
== system CAProcessorInTheLoop/Plant/Road Inclination Tests/Plug ==
  In1 : Inport
  Out1 : Outport
  wires:
  In1/1 -> Out1/1

== matlab function CAProcessorInTheLoop/MATLAB Function1 ==
  data: Speed input; y output; Sign input; max_speed_fw input; max_speed_bw input
function y = SpeedEval(Speed, Sign, max_speed_fw, max_speed_bw)
if(Sign==1) % positive speed
    y = Speed*max_speed_fw/5;
else
    y = -Speed*max_speed_bw/5;
end

== matlab function CAProcessorInTheLoop/MATLAB Function ==
  data: P input; ATS output int8; R input; N input; D input; B input
function ATS = Bits2AutomaticTransmissionState(P, R, N, D, B)
if(P==1 && R==0 && N==0 && D==0 && B==0) % Park
    ATS = 0;
elseif (P==0 && R==1 && N==0 && D==0 && B==0) % Reverse
    ATS = 1;
elseif (P==0 && R==0 && N==1 && D==0 && B==0) % Neutral
    ATS = 2;
elseif (P==0 && R==0 && N==0 && D==1 && B==0) % Drive
    ATS = 3;
elseif (P==0 && R==0 && N==0 && D==0 && B==1) % Brake
    ATS = 4;
else
    ATS = -1; % Generates SW error
end
ATS=int8(ATS);
end

== matlab function CAProcessorInTheLoop/MATLAB Function2 ==
  data: ATS input; P output boolean; R output boolean; N output boolean; D output boolean; B output boolean
function [P,R,N,D,B] = AutomaticTransmissionState2Bits(ATS)
P = false;
R = false;
N = false;
D = false;
B = false;
switch ATS
    case 0
        P = true;
    case 1
        R = true;
    case 2
        N = true;
    case 3
        D = true;
    case 4
        B = true;
end

== stateflow chart CAProcessorInTheLoop/Subsystem/Blinker ==
  state Initial
  state On
    entry:
    out=true;
  state Blink
  state Off
    entry:
    out=false;
  (default) -> Initial
  Initial -> On : [inp==true]
  On -> Blink : [inp==false]
  Blink -> Off : [after(5,sec)]
  (junction 10) -> Initial
  Off -> (junction 9)
  (junction 9) -> (junction 10)
  data: inp input; out output

== stateflow chart CAProcessorInTheLoop/Subsystem/Blinker1 ==
  state Initial
  state On
    entry:
    out=true;
  state Blink
  state Off
    entry:
    out=false;
  (default) -> Initial
  Initial -> On : [inp==true]
  On -> Blink : [inp==false]
  Blink -> Off : [after(5,sec)]
  (junction 10) -> Initial
  Off -> (junction 9)
  (junction 9) -> (junction 10)
  data: inp input; out output

== stateflow chart CAProcessorInTheLoop/Subsystem/Blinker2 ==
  state Initial
  state On
    entry:
    out=true;
  state Blink
  state Off
    entry:
    out=false;
  (default) -> Initial
  Initial -> On : [inp==true]
  On -> Blink : [inp==false]
  Blink -> Off : [after(5,sec)]
  (junction 10) -> Initial
  Off -> (junction 9)
  (junction 9) -> (junction 10)
  data: inp input; out output

== stateflow chart CAProcessorInTheLoop/Subsystem/CAN Analyzer ==
  note: CANbus fault analyzer
  state Working
    entry:
    lightCANbusFailure=false;
    canbusFault=false;
  state NoSignal
  note: For better safety, the fault can be
      | resetted only by restarting the car,
      | even if the CANbus becomes functioning
      | again during use
  state Fault
    entry:
    lightCANbusFailure=true;
    canbusFault=true;
  (default) -> Working
  Working -> NoSignal : [canbusDataStatus==0]
  NoSignal -> Working [order 1] : [canbusDataStatus==1]
  NoSignal -> Fault [order 2] : after(FAULT_TOLERANCE_TIME,msec)
  data: canbusFault output boolean; canbusDataStatus input; FAULT_TOLERANCE_TIME constant double =300; lightCANbusFailure output boolean =false

== matlab function CAProcessorInTheLoop/Subsystem/RedundantTPPSensorsChecker/MATLAB Function ==
  data: sensor1 input single; errorFlag output; sensor2 input single; sensor3 input single; selected output single; not_selected output single
function [errorFlag, selected, not_selected] = selectSensors(sensor1, sensor2, sensor3)
    errorFlag = true;
    if sensor1 == sensor2 && sensor2 == sensor3
        selected = sensor1;
        not_selected = single(-1);
        errorFlag = false;
    elseif sensor1 == sensor2
        selected = sensor1;
        not_selected = sensor3;
    elseif sensor2 == sensor3
        selected = sensor2;
        not_selected = sensor1;
    else
        selected = sensor3;
        not_selected = sensor2;
    end
end

== stateflow chart CAProcessorInTheLoop/Subsystem/Transmission and Torque Controller ==
  state brakeLightToggle [function]
    (default) -> (junction 215) : % LightToggle
    (junction 215) -> (junction 216) [order 1] : [lightPressBrake==true&&brakePedalPressed==1]
    (junction 215) -> (junction 217) [order 2]
    (junction 216) -> (junction 218) : {lightPressBrake=false;}
    (junction 218) -> (junction 217)
    (junction 217) -> (junction 219)
  state starting(speedValue) [function]
    (default) -> (junction 64) : % BrakeReselasedCheck
    (junction 64) -> (junction 65) [order 1] : [brakePedalPressed==0]
    (junction 64) -> (junction 66) [order 2] : {desiredSpeed_km_h=0;}
    (junction 65) -> (junction 67) : {desiredSpeed_km_h=speedValue;}
    (junction 67) -> (junction 66)
    (junction 66) -> (junction 68)
  note: Transmission and Torque Controller
  state Working
    entry:
    lightTppSensorFailure=false;
    lightMaxTorqueLimited=false;
    lightSWFailure=false;
    state Park
      entry:
      automaticTransmissionState=Park;
      %activate EHandbrake
      during:
      brakeControllerEnable=false;
      desiredTorque_Nm=0;
    state Neutral
      entry:
      automaticTransmissionState=Neutral;
      startingControllerEnable=false;
      during:
      desiredTorque_Nm=0;
      brakeControllerEnable=false;
    state Drive
      entry:
      automaticTransmissionState=Drive;
      startingControllerEnable=false;
      lightAutomaticGC=false;
      lightBatteryTooHigh=false;
      during:
      desiredTorque_Nm=throttlePedalPosition*MAX_TORQUE;
      brakeLightToggle()
      state Driving
        during:
        brakeControllerEnable=false;
      state StopAndStart
        entry:
        %activate EHandbrake
        during:
        startingControllerEnable=true;
        starting(STARTING_SPEED)
        exit:
        startingControllerEnable=false;
      (default) -> Driving
      Driving -> Working.Drive.StopAndStart : [abs(vehicleSpeed_km_h)<=0.5&&brakePedalPressed==true&&canbusFault~=1]
      Working.Drive.StopAndStart -> Driving [order 1] : [throttlePedalPosition~=0&&brakePedalPressed==false]
      Working.Drive.StopAndStart -> Driving [order 3] : [canbusFault==1]{lightPressBrake=true;}
      Working.Drive.StopAndStart -> Driving [order 2] : [vehicleSpeed_km_h>STARTING_SPEED+1]{lightPressBrake=true;}
    state Brake
      entry:
      automaticTransmissionState=Brake;
      startingControllerEnable=false;
      during:
      brakeLightToggle()
      state RegenerativeBraking
        during:
        desiredTorque_Nm=-MAX_TORQUE_REVERSE*(1-3*throttlePedalPosition);
        desiredSpeed_km_h=0;
        lightPressBrake=false;
        brakeControllerEnable=true;
      state Acceleration
        during:
        desiredTorque_Nm=MAX_TORQUE*3/2*(throttlePedalPosition-1/3);
        brakeControllerEnable=false;
      state StopAndStart
        entry:
        %activate EHandbrake
        during:
        desiredTorque_Nm=-MAX_TORQUE*(1-3*throttlePedalPosition);
        startingControllerEnable=true;
        starting(STARTING_SPEED)
        exit:
        startingControllerEnable=true;
      (default) -> Acceleration
      Acceleration -> RegenerativeBraking : [throttlePedalPosition<1/3]
      RegenerativeBraking -> Acceleration [order 1] : [throttlePedalPosition>=1/3]
      RegenerativeBraking -> Working.Brake.StopAndStart [order 2] : [abs(vehicleSpeed_km_h)<=0.5&&brakePedalPressed==true]
      Working.Brake.StopAndStart -> RegenerativeBraking [order 2] : [vehicleSpeed_km_h>STARTING_SPEED+1]
          | {lightPressBrake=true;}
      (junction 72) -> Acceleration
      Working.Brake.StopAndStart -> (junction 72) [order 1] : [throttlePedalPosition>=1/3&&brakePedalPressed==false]
    state Reverse
      entry:
      automaticTransmissionState=Reverse;
      during:
      desiredTorque_Nm=-throttlePedalPosition*MAX_TORQUE_REVERSE;
      brakeControllerEnable=false;
    Working.Drive -> Working.Drive [order 3] : [automaticTrasmissionSelectorState==4&&throttlePedalPosition>1/3&&batteryChargeValue>BATTERY_SAFE_LEVEL_PERCENTAGE]
        | {lightBatteryTooHigh=true;}
    Working.Drive -> Working.Drive [order 2] : [automaticTrasmissionSelectorState==4&&canbusFault==1]
    (default) -> Working.Neutral
    Working.Neutral -> Working.Drive [order 1] : [automaticTrasmissionSelectorState>=3&&brakePedalPressed==true&&vehicleSpeed_km_h>-5]
    Working.Neutral -> Working.Park [order 2] : [automaticTrasmissionSelectorState==0&&brakePedalPressed==true&&abs(vehicleSpeed_km_h)<=5]
    Working.Park -> Working.Neutral : [automaticTrasmissionSelectorState~=0&&brakePedalPressed==true]
    Working.Drive -> Working.Neutral [order 1] : [automaticTrasmissionSelectorState<3]
    Working.Neutral -> Working.Reverse [order 3] : [automaticTrasmissionSelectorState==1&&brakePedalPressed==true&&vehicleSpeed_km_h<=5]
    Working.Reverse -> Working.Neutral : [automaticTrasmissionSelectorState~=1]
    Working.Drive -> Brake [order 4] : [automaticTrasmissionSelectorState==4&&throttlePedalPosition>1/3]
    Brake -> Working.Drive [order 1] : [automaticTrasmissionSelectorState~=4]
    Brake -> Working.Drive [order 2] : [canbusFault==1]{lightAutomaticGC=true;}
  state LimpHomeMode
    entry:
    brakeControllerEnable=false;
    startingControllerEnable=false;
    lightTppSensorFailure=true;
    lightMaxTorqueLimited=true;
    state EntryTransitionState
    state Park
      entry:
      automaticTransmissionState=Park;
      %activate EHandbrake
      during:
      desiredTorque_Nm=0;
    state Neutral
      entry:
      automaticTransmissionState=Neutral;
      during:
      desiredTorque_Nm=0;
    state Drive
      entry:
      automaticTransmissionState=Drive;
      during:
      desiredTorque_Nm=throttlePedalPosition*MAX_TORQUE_FAULT;
      lightAutomaticGC=false;
    state Reverse
      entry:
      automaticTransmissionState=Reverse;
      during:
      desiredTorque_Nm=-throttlePedalPosition*MAX_TORQUE_FAULT;
    (default) -> EntryTransitionState
    EntryTransitionState -> (junction 152) [order 2] : [automaticTransmissionState==Reverse]
    (junction 152) -> (junction 153)
    EntryTransitionState -> (junction 158) [order 4] : [automaticTransmissionState==Drive]
    EntryTransitionState -> (junction 143) [order 1] : [automaticTransmissionState==Park]
    (junction 158) -> LimpHomeMode.Drive
    (junction 143) -> LimpHomeMode.Park
    EntryTransitionState -> (junction 144) [order 3] : [automaticTransmissionState==Brake]{lightAutomaticGC=true}
    (junction 144) -> LimpHomeMode.Drive
    EntryTransitionState -> LimpHomeMode.Neutral [order 5]
    LimpHomeMode.Neutral -> LimpHomeMode.Drive [order 2] : [automaticTrasmissionSelectorState>=3&&brakePedalPressed==true&&vehicleSpeed_km_h>-5]
    LimpHomeMode.Neutral -> LimpHomeMode.Park [order 1] : [automaticTrasmissionSelectorState==0&&brakePedalPressed==true&&abs(vehicleSpeed_km_h)<=5]
    LimpHomeMode.Drive -> LimpHomeMode.Neutral : [automaticTrasmissionSelectorState<3]
    LimpHomeMode.Park -> LimpHomeMode.Neutral : [automaticTrasmissionSelectorState~=0&&brakePedalPressed==true]
    LimpHomeMode.Neutral -> LimpHomeMode.Reverse [order 3] : [automaticTrasmissionSelectorState==1&&brakePedalPressed==true&&vehicleSpeed_km_h<=5]
    LimpHomeMode.Reverse -> LimpHomeMode.Neutral : [automaticTrasmissionSelectorState~=1]
    (junction 153) -> LimpHomeMode.Reverse
  note: Note that disp("message") indicates that a warning light should turn on in the dashboard with that related meaning (plus, when needed, a sound alarm should sounds too, as indicated in the pdf document).
  note: The reset constant emulate a software reset via canbus after the car has been repaired correctly. This option cannot be done by the driver and has to be done by a certified mechanic
  state SoftwareFailurePlausibilityCheck
    entry:
    lightSWFailure=true;
    startingControllerEnable=false;
    brakeControllerEnable=false;
    state Neutral
      entry:
      automaticTransmissionState=Neutral;
      during:
      desiredTorque_Nm=0;
    state HotSwap
      %hotswap CPU
    (default) -> HotSwap
    HotSwap -> SoftwareFailurePlausibilityCheck.Neutral : %if hotswap fails
  (default) -> Working
  LimpHomeMode -> Working : [reset==1]
  Working -> LimpHomeMode [order 1] : [ttpSensorFault==1]
  SoftwareFailurePlausibilityCheck -> Working : [reset==1]
  Working -> SoftwareFailurePlausibilityCheck [order 2] : [automaticTrasmissionSelectorState>4||automaticTrasmissionSelectorState<0||vehicleSpeed_km_h>MAX_SPEED_FORWARD...
      | ||vehicleSpeed_km_h<-MAX_SPEED_BACKWARD||throttlePedalPosition>1||throttlePedalPosition<0]
  data: speedValue function_input; automaticTransmissionState output Enum: TransmissionState; throttlePedalPosition input single; ttpSensorFault input; brakePedalPressed input; automaticTrasmissionSelectorState input; canbusFault input; batteryChargeValue input; vehicleSpeed_km_h input; MAX_TORQUE parameter single size=1; desiredTorque_Nm output single; brakeControllerEnable output; startingControllerEnable output; MAX_TORQUE_REVERSE parameter single size=1; desiredSpeed_km_h output single; STARTING_SPEED constant single =3; MAX_TORQUE_FAULT local =35; BATTERY_SAFE_LEVEL_PERCENTAGE constant single =90; MAX_SPEED_BACKWARD parameter; MAX_SPEED_FORWARD parameter; reset input =0; lightSWFailure output boolean =false; lightPressBrake output boolean =false; lightBatteryTooHigh output boolean =false; lightMaxTorqueLimited output boolean =false; lightTppSensorFailure output boolean =false; lightAutomaticGC output boolean =false
